simulink model "S4_ESC_Lab"  (R2025b)
settings: Solver=ode23t  StartTime=0.0  StopTime=inf  MaxStep=maxStep  RelTol=1e-4
values from neighbouring files (symbols this model uses):
  MF = [4 2.0 0.10 1.00]    [ABS_Utils.m]
undefined symbols (not defined in the file or in its folder): g, Jmax, Jmin, k, KiSlip, KpSlip, lambdaMax, lambdaMin, mode, mq, objectiveGain, Rw, stopV, Tmax, Tmin, Topen
libraries: nesl_utility x8, fl_lib x7, simulink x2, slctrl_adaptive x1, sdl_lib x1
settings Model: Creator=leffe  LastModifiedBy=leffe
settings OptimizationCC: BlockReduction=off  OptimizeBlockIOStorage=off

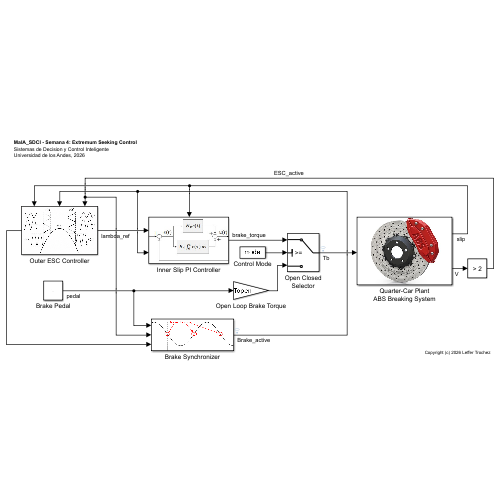
[thumbnail: Simulink's stored preview of the top-level diagram]
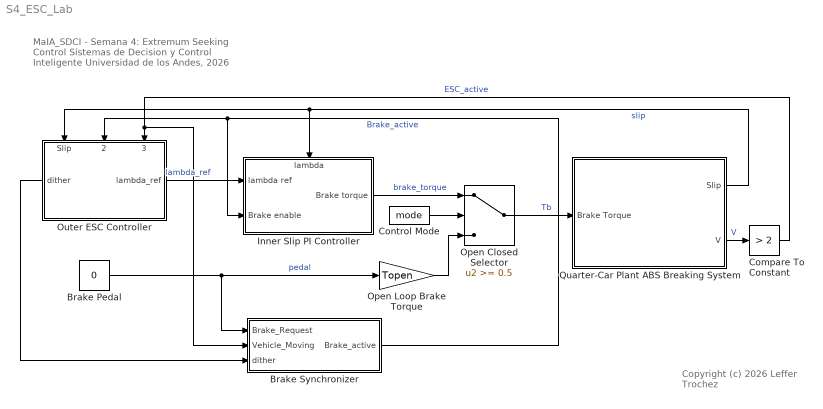
== system S4_ESC_Lab ==
  note: Copyright (c) 2026 Leffer Trochez
  note: MaIA_SDCI - Semana 4: Extremum Seeking Control
      | Sistemas de Decision y Control Inteligente
      | Universidad de los Andes, 2026
  Brake Pedal : Constant  Value=0  SampleTime=0
  Brake Synchronizer : Subsystem
      mask Display: image('hit crossing.png');
  Compare To Constant : simulink/Logic and Bit Operations/Compare To Constant  relop=>  const=2  OutDataTypeStr=boolean
  Control Mode : Constant  Value=mode
  Inner Slip PI Controller : Subsystem
      settings: PortSchema="{\"entries\":[{\"content\":{\"sides\":[{\"content\":{\"connectorIds\":[\"In1\",\"In2\"]},\"type\":\"ConnectorPlacement.EquallySpacedRectSide\",\"uuid\":\"2d8152cb-e1e7-4cbd-90d9-1ad452f9118c\"},{\"content\":{\"connectorIds\":[\"Out1\"],\"side\":\"RIGHT\"},\"type\":\"ConnectorPlacement.EquallySpacedRectSide\",\"uuid\":\"1543b6c9-e8db-48f7-9c77-f5e8a9c4fad1\"},{\"content\":{\"connectorIds\":[\"In3\"],\"side\":\"TOP\"},\"type\":\"ConnectorPlacement.EquallySpacedRectSide\",\"uuid\":\"3b9f2303-2b56-4e0e-9eaf-6ad78f3600f9\"}]},\"type\":\"ConnectorPlacement.EquallySpacedConnector\",\"uuid\":\"5e2a5701-87ef-4f6c-be32-195e55163038\"}],\"packageUris\":[\"http://schema.mathworks.com/mf0/Connector/R2020b\"],\"version\":\"1.0\"}"
      mask Display: image('PI.jpg');
  Open Closed Selector : Switch  Threshold=0.5  SaturateOnIntegerOverflow=off  InputSameDT=off
  Open Loop Brake Torque : Gain  Gain=Topen
  Outer ESC Controller : Subsystem
      settings: PortSchema="{\"entries\":[{\"content\":{\"sides\":[{\"content\":{\"connectorIds\":[\"Out2\"]},\"type\":\"ConnectorPlacement.EquallySpacedRectSide\",\"uuid\":\"31de49aa-46d4-4a9a-8690-efbb2b420d0d\"},{\"content\":{\"connectorIds\":[\"Out1\"],\"side\":\"RIGHT\"},\"type\":\"ConnectorPlacement.EquallySpacedRectSide\",\"uuid\":\"18edca33-0aae-4427-96c8-3219eae31a8b\"},{\"content\":{\"connectorIds\":[\"In1\",\"In2\",\"In3\"],\"side\":\"TOP\"},\"type\":\"ConnectorPlacement.EquallySpacedRectSide\",\"uuid\":\"43769023-76ac-4312-8342-8169355bc34d\"}]},\"type\":\"ConnectorPlacement.EquallySpacedConnector\",\"uuid\":\"6a090688-03d4-4148-bdef-ff5198eebe00\"}],\"packageUris\":[\"http://schema.mathworks.com/mf0/Connector/R2020b\"],\"version\":\"1.0\"}"
      mask Display: image('ESC.png');
  Quarter-Car Plant ABS Breaking System : Subsystem
      mask Display: image('ABS.jpg');
  wires:
  Brake Pedal/1 -> Brake Synchronizer/1(Brake_Request), Open Loop Brake Torque/1  "pedal"
  Inner Slip PI Controller/1(Brake torque) -> Open Closed Selector/1  "brake_torque"
  Quarter-Car Plant ABS Breaking System/1(Slip) -> Outer ESC Controller/1(Slip), Inner Slip PI Controller/3(lambda)  "slip"
  Open Loop Brake Torque/1 -> Open Closed Selector/3
  Control Mode/1 -> Open Closed Selector/2
  Open Closed Selector/1 -> Quarter-Car Plant ABS Breaking System/1(Brake Torque)  "Tb"
  Outer ESC Controller/1(lambda_ref) -> Inner Slip PI Controller/1(lambda ref)  "lambda_ref"
  Quarter-Car Plant ABS Breaking System/2(V) -> Compare To Constant/1  "V"
  Compare To Constant/1 -> Outer ESC Controller/3(ESC_active), Brake Synchronizer/2(Vehicle_Moving)  "ESC_active"
  Brake Synchronizer/1(Brake_active) -> Inner Slip PI Controller/2(Brake enable), Outer ESC Controller/2(Brake_active)  "Brake_active"
  Outer ESC Controller/2(dither) -> Brake Synchronizer/3(dither)

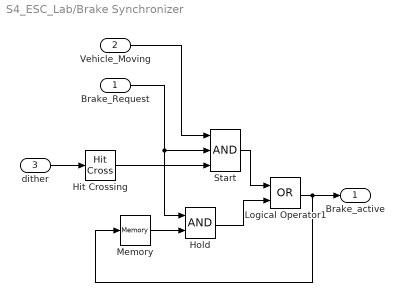
== system S4_ESC_Lab/Brake Synchronizer ==
  Brake_Request : Inport
  Vehicle_Moving : Inport  Port=2
  dither : Inport  Port=3
  Hit Crossing : HitCross  HitCrossingDirection=rising
  Hold : Logic  AllPortsSameDT=off  OutDataTypeStr=boolean
  Logical Operator1 : Logic  Operator=OR  AllPortsSameDT=off  OutDataTypeStr=boolean
  "Memory " : Memory
  Start : Logic  Inputs=3  AllPortsSameDT=off  OutDataTypeStr=boolean
  Brake_active : Outport
  wires:
  dither/1 -> Hit Crossing/1
  Brake_Request/1 -> Hold/1, Start/2
  Vehicle_Moving/1 -> Start/1
  Hit Crossing/1 -> Start/3
  "Memory "/1 -> Hold/2
  Start/1 -> Logical Operator1/1
  Hold/1 -> Logical Operator1/2
  Logical Operator1/1 -> "Memory "/1, Brake_active/1

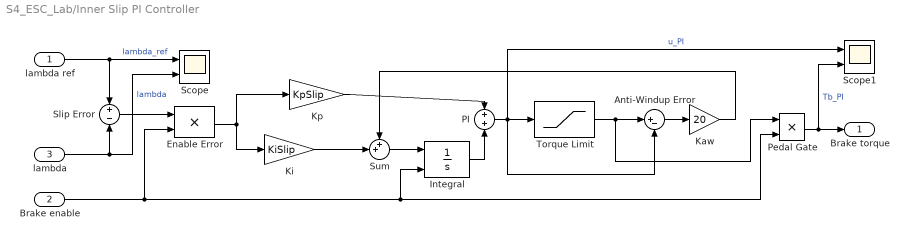
== system S4_ESC_Lab/Inner Slip PI Controller ==
  lambda ref : Inport
  Brake enable : Inport  Port=2
  lambda : Inport  Port=3
  Anti-Windup Error : Sum  Inputs=|+-
  Enable Error : Product  Inputs=**
  Integral : Integrator  ExternalReset=falling  LimitOutput=on  UpperSaturationLimit=Tmax  LowerSaturationLimit=0
  Kaw : Gain  Gain=20
  Ki : Gain  Gain=KiSlip
  Kp : Gain  Gain=KpSlip
  PI : Sum
  Pedal Gate : Product  Inputs=**
  Scope : Scope  NumInputPorts=2
      settings: ActiveDisplayYMinimum=-0.024789664527761449  ActiveDisplayYMaximum=0.22310698074985311
  Scope1 : Scope  NumInputPorts=2
      settings: ActiveDisplayYMinimum=-525.00598935884784  ActiveDisplayYMaximum=4725.0539042296314
  Slip Error : Sum  Inputs=+-
  Sum : Sum  Inputs=++|
  Torque Limit : Saturate  UpperLimit=Tmax  LowerLimit=Tmin
  Brake torque : Outport
  wires:
  Slip Error/1 -> Enable Error/1
  Brake enable/1 -> Enable Error/2, Pedal Gate/2, Integral/2
  Enable Error/1 -> Kp/1, Ki/1
  Kp/1 -> PI/1
  Integral/1 -> PI/2
  PI/1 -> Anti-Windup Error/2, Scope1/1, Torque Limit/1  "u_PI"
  Pedal Gate/1 -> Brake torque/1, Scope1/2  "Tb_PI"
  lambda ref/1 -> Slip Error/1, Scope/1  "lambda_ref"
  lambda/1 -> Slip Error/2, Scope/2  "lambda"
  Torque Limit/1 -> Anti-Windup Error/1, Pedal Gate/1
  Anti-Windup Error/1 -> Kaw/1
  Sum/1 -> Integral/1
  Ki/1 -> Sum/2
  Kaw/1 -> Sum/1

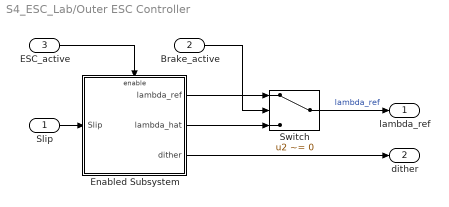
== system S4_ESC_Lab/Outer ESC Controller ==
  Slip : Inport
  Brake_active : Inport  Port=2
  ESC_active : Inport  Port=3
  "Enabled Subsystem " : Subsystem  TreatAsAtomicUnit=on
  Switch : Switch  Criteria=u2 ~= 0  SaturateOnIntegerOverflow=off  InputSameDT=off
  lambda_ref : Outport
  dither : Outport  Port=2
  wires:
  Slip/1 -> "Enabled Subsystem "/1(Slip)
  "Enabled Subsystem "/1(lambda_ref) -> Switch/1
  Brake_active/1 -> Switch/2
  "Enabled Subsystem "/2(lambda_hat) -> Switch/3
  Switch/1 -> lambda_ref/1  "lambda_ref"
  "Enabled Subsystem "/3(dither) -> dither/1
  ESC_active/1 -> "Enabled Subsystem "/Enable

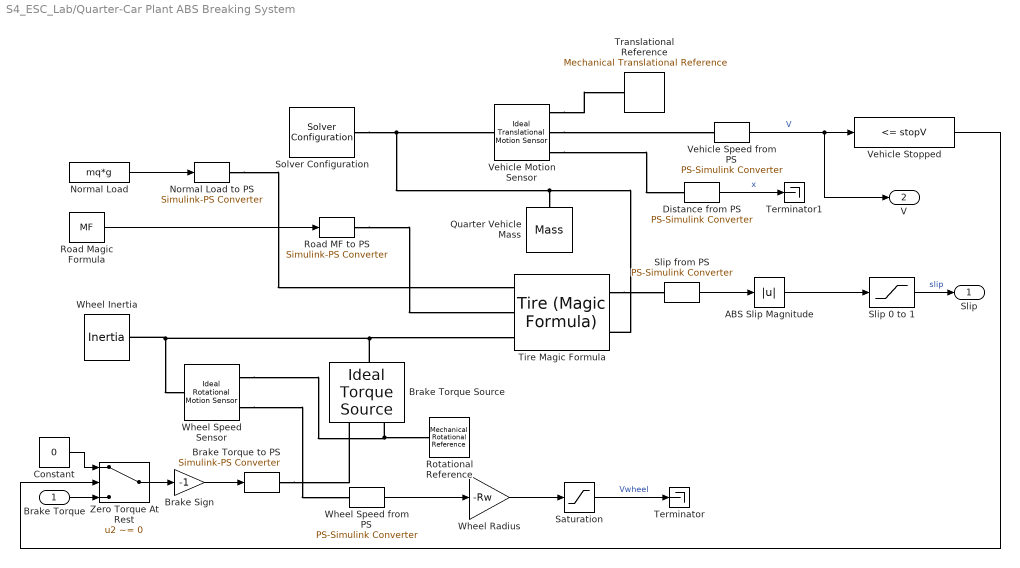
== system S4_ESC_Lab/Quarter-Car Plant ABS Breaking System ==
  Brake Torque : Inport
  ABS Slip Magnitude : Abs  SaturateOnIntegerOverflow=off
  Brake Sign : Gain  Gain=-1
  Brake Torque Source : fl_lib/Mechanical/Mechanical Sources/Ideal Torque Source
  Brake Torque to PS : nesl_utility/Simulink-PS Converter  PhysicalDomain=network_engine_domain  SubClassName=ps_input  LeftPortType=input  RightPortType=output  PseudoPeriodic=off  Frequencies=[]  NoiseDistribution=none  NoiseParameters=[]  Unit=N*m  AffineConversion=off  FilteringAndDerivatives=provide  SimscapeFilterOrder=1  InputFilterTimeConstant=0.001  UdotUserProvided=0
  Constant : Constant  Value=0
  Distance from PS : nesl_utility/PS-Simulink Converter  PhysicalDomain=network_engine_domain  SubClassName=ps_output  LeftPortType=input  RightPortType=output  PseudoPeriodic=off  Frequencies=[]  VectorFormat=inherit  Unit=m  AffineConversion=off
  Normal Load : Constant  Value=mq*g
  Normal Load to PS : nesl_utility/Simulink-PS Converter  PhysicalDomain=network_engine_domain  SubClassName=ps_input  LeftPortType=input  RightPortType=output  PseudoPeriodic=off  Frequencies=[]  NoiseDistribution=none  NoiseParameters=[]  Unit=N  AffineConversion=off  FilteringAndDerivatives=provide  SimscapeFilterOrder=1  InputFilterTimeConstant=0.001  UdotUserProvided=0
  Quarter Vehicle Mass : fl_lib/Mechanical/Translational Elements/Mass  mass=mq kg  num_ports=foundation.enum.numPorts2.one  v_specify=on  v_priority=High  v=v0 m/s  v_nominal_specify=off  v_nominal_value=1  v_nominal_unit=m/s  f_specify=off  f_priority=None  f=0 N  f_nominal_specify=off  f_nominal_value=1  f_nominal_unit=N
  Road MF to PS : nesl_utility/Simulink-PS Converter  PhysicalDomain=network_engine_domain  SubClassName=ps_input  LeftPortType=input  RightPortType=output  PseudoPeriodic=off  Frequencies=[]  NoiseDistribution=none  NoiseParameters=[]  Unit=1  AffineConversion=off  FilteringAndDerivatives=provide  SimscapeFilterOrder=1  InputFilterTimeConstant=0.001  UdotUserProvided=0
  Road Magic Formula : Constant  Value=MF
  Rotational Reference : fl_lib/Mechanical/Rotational Elements/Mechanical Rotational Reference
  Saturation : Saturate  UpperLimit=0  LowerLimit=-inf
  Slip 0 to 1 : Saturate  UpperLimit=1  LowerLimit=0
  Slip from PS : nesl_utility/PS-Simulink Converter  PhysicalDomain=network_engine_domain  SubClassName=ps_output  LeftPortType=input  RightPortType=output  PseudoPeriodic=off  Frequencies=[]  VectorFormat=inherit  Unit=1  AffineConversion=off
  Solver Configuration : nesl_utility/Solver Configuration  PhysicalDomain=network_engine_domain  SubClassName=solver  LeftPortType=input  RightPortType=generic  Tones=[]  Harmonics=[]  SimulateNoise=off  Profile=off  UseLocalSampling=off  EnableSwitchedLinearOptims=on  FrequencyDomain=off  UseCCode=off  RelTol=0.001  AbsTol=0.001  MinStep=1e-09  ToWorkspace=off  RevertToSquareIcSolve=off  NumHomotopyIterations=100  PhasorMode=off  PhasorModeNumHarmonics=1  ConsistencySolver=NEWTON_XTOL_AFTER_FTOL  IndexReductionMethod=DerivativeReplacement  DoDC=off  ResidualTolerance=1e-09  ConsistencyTolSource=GLOBAL  ConsistencyAbsTol=0.001  ConsistencyRelTol=0.001  ConsistencyTolFactor=0.001  UseLocalSolver=off  LocalSolverChoice=NE_BACKWARD_EULER_ADVANCER  ResolveIndetEquations=on  FunctionEvalNumThread=1  LocalSolverSampleTime=0.001  DoFixedCost=off  MaxNonlinIter=3  MaxModeIter=2  ComputeImpulses=off  ImpulseIterations=2  LinearAlgebra=auto  LinearAlgebraNumThread=0  EquationFormulation=NE_TIME_EF  DelaysMemoryBudget=1024  AutomaticFiltering=on  FilteringTimeConstant=0.001  PartitionStorageMethod=AS_NEEDED  PartitionMemoryBudget=1024  PartitionMethod=ROBUST  MultibodyUseLocalSolver=off  MultibodyLocalSolverChoice=ODE1  MultibodyLocalSolverSampleTime=0.001
  Terminator : Terminator
  Terminator1 : Terminator
  Tire Magic Formula : sdl_lib/Tires & Vehicles/Tire (Magic Formula)  parameterization=sdl.enum.magic_tire_model.PS  F_z1=3000 N  F_x1=3500 N  kappa1=10  B_m=10  C_m=1.9  D_m=1  E_m=0.97  fz0=4000 N  p_Cx=1.685  p_Dx=[1.21, -.037]  p_Ex=[.344, .095, -.02, 0]  p_Kx=[21.51, -.163, .245]  p_Hx=[-.002, .002]  p_Vx=[0, 0]  rolling_radius_model=sdl.enum.RollingRadiusParameterization.Constant  r_e=Rw m  r_0=0.3 m  breff=8.39  dreff=0.26  freff=0.074  q_re0=0.99  q_v1=0.008  longvl=17 m/s  cz=5e5 N/m  model_resistance=0  resistance_model=sdl.enum.rollingResistanceParameterization.constant  coeff=0.015  p_tire=250e3 Pa  alpha=-0.003  beta=0.97  coeff_a=84e-4  coeff_b=6.2e-4 s/m  coeff_c=1.6e-4 s^2/m^2  p_tire0=240e3 Pa  fz0_resistance=4000 N  vH0=16 m/s  q_Sy=[.0082, 0, .0014, .001, 0, 0, 1.08, -.5]  v_thr=0.001 m/s  enable_scaling_coefficients=false  lfzO=1  lcx=1  lmux=1  lex=1  lkx=1  lhx=1  lvx=1  lmy=1  model_compliance=0  stiffness=1e6 N/m  damping=1000 N*s/m  model_inertia=0  inertia=1 kg*m^2  initial_velocity=0 rad/s  vxlow=1 m/s  v_tr_thr=0.1 m/s  kpumin=-1.5  kpumax=1.5
      settings: InternalSimscapePortConfiguration="{\"Bottom\":[],\"Left\":[{\"id\":\"N\",\"label\":\"N\",\"type\":\"input\"},{\"id\":\"M\",\"label\":\"M\",\"type\":\"input\"},{\"id\":\"A\",\"label\":\"A\",\"type\":\"foundation.mechanical.rotational.rotational\"}],\"Right\":[{\"id\":\"S\",\"label\":\"S\",\"type\":\"output\"},{\"id\":\"H\",\"label\":\"H\",\"type\":\"foundation.mechanical.translational.translational\"}],\"Top\":[]}"
  Translational Reference : fl_lib/Mechanical/Translational Elements/Mechanical Translational Reference
  Vehicle Motion Sensor : fl_lib/Mechanical/Mechanical Sensors/Ideal Translational Motion Sensor  reference=foundation.enum.MeasurementReference.difference  acceleration_port=false  velocity_port=true  position_port=true  offset=0 m
  Vehicle Speed from PS : nesl_utility/PS-Simulink Converter  PhysicalDomain=network_engine_domain  SubClassName=ps_output  LeftPortType=input  RightPortType=output  PseudoPeriodic=off  Frequencies=[]  VectorFormat=inherit  Unit=m/s  AffineConversion=off
  Vehicle Stopped : simulink/Logic and Bit Operations/Compare To Constant  relop=<=  const=stopV  OutDataTypeStr=boolean
  Wheel Inertia : fl_lib/Mechanical/Rotational Elements/Inertia  inertia=Jw kg*m^2  num_ports=foundation.enum.numPorts2.one  w_specify=on  w_priority=High  w=w0 rad/s  w_nominal_specify=off  w_nominal_value=1  w_nominal_unit=rad/s  t_specify=off  t_priority=None  t=0 N*m  t_nominal_specify=off  t_nominal_value=1  t_nominal_unit=N*m
  Wheel Radius : Gain  Gain=-Rw
  Wheel Speed Sensor : fl_lib/Mechanical/Mechanical Sensors/Ideal Rotational Motion Sensor  reference=foundation.enum.MeasurementReference.difference  acceleration_port=false  velocity_port=true  position_port=false  wrap_angle=false  offset=0 rad
      settings: InternalSimscapePortConfiguration="{\"Bottom\":[],\"Left\":[{\"id\":\"R\",\"label\":\"R\",\"type\":\"foundation.mechanical.rotational.rotational\"}],\"Right\":[{\"id\":\"C\",\"label\":\"C\",\"type\":\"foundation.mechanical.rotational.rotational\"},{\"id\":\"W\",\"label\":\"W\",\"type\":\"output\"}],\"Top\":[]}"
  Wheel Speed from PS : nesl_utility/PS-Simulink Converter  PhysicalDomain=network_engine_domain  SubClassName=ps_output  LeftPortType=input  RightPortType=output  PseudoPeriodic=off  Frequencies=[]  VectorFormat=inherit  Unit=rad/s  AffineConversion=off
  Zero Torque At Rest : Switch  Criteria=u2 ~= 0  SaturateOnIntegerOverflow=off  InputSameDT=off
  Slip : Outport
  V : Outport  Port=2
  wires:
  Normal Load/1 -> Normal Load to PS/1
  Road Magic Formula/1 -> Road MF to PS/1
  Wheel Speed from PS/1 -> Wheel Radius/1
  Slip from PS/1 -> ABS Slip Magnitude/1
  Distance from PS/1 -> Terminator1/1  "x"
  ABS Slip Magnitude/1 -> Slip 0 to 1/1
  Slip 0 to 1/1 -> Slip/1  "slip"
  Vehicle Speed from PS/1 -> V/1, Vehicle Stopped/1  "V"
  Vehicle Stopped/1 -> Zero Torque At Rest/2
  Constant/1 -> Zero Torque At Rest/1
  Brake Torque/1 -> Zero Torque At Rest/3
  Wheel Radius/1 -> Saturation/1
  Zero Torque At Rest/1 -> Brake Sign/1
  Brake Sign/1 -> Brake Torque to PS/1
  Saturation/1 -> Terminator/1  "Vwheel"
  connections:
  Brake Torque to PS/RConn1 -- Brake Torque Source/RConn1
  Wheel Speed Sensor/RConn1 -- Brake Torque Source/RConn2 -- Rotational Reference/LConn1
  Wheel Speed Sensor/RConn2 -- Wheel Speed from PS/LConn1
  Normal Load to PS/RConn1 -- Tire Magic Formula/LConn1
  Solver Configuration/RConn1 -- Tire Magic Formula/RConn2 -- Quarter Vehicle Mass/LConn1 -- Vehicle Motion Sensor/LConn1
  Road MF to PS/RConn1 -- Tire Magic Formula/LConn2
  Brake Torque Source/LConn1 -- Wheel Speed Sensor/LConn1 -- Wheel Inertia/LConn1 -- Tire Magic Formula/LConn3
  Vehicle Motion Sensor/RConn2 -- Vehicle Speed from PS/LConn1
  Vehicle Motion Sensor/RConn1 -- Translational Reference/LConn1
  Vehicle Motion Sensor/RConn3 -- Distance from PS/LConn1
  Tire Magic Formula/RConn1 -- Slip from PS/LConn1

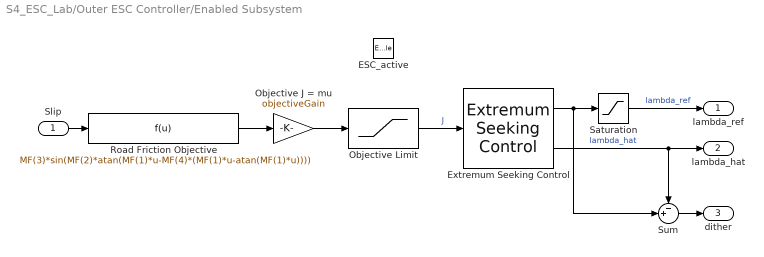
== system S4_ESC_Lab/Outer ESC Controller/Enabled Subsystem  ==
  Slip : Inport
  ESC_active : EnablePort
  " Saturation " : Saturate  UpperLimit=lambdaMax  LowerLimit=lambdaMin
  "Extremum Seeking Control " : slctrl_adaptive/Extremum Seeking Control  timeDomainStatus=Continuous time  SampleTime=0.1  IntegratorMethods=Forward Euler  paramCount=1  initialVal=lambda0  omega=omega  gain=k  demodAmp=demodAmp  demodPhase=demodPhase  modAmp=b  modPhase=modPhase  highPassEnable=on  highPassCutoff=wh  lowPassEnable=on  lowPassCutoff=wl  estimatedVarOn=on  HPFFreq=1  LPFFreq=2  SampleTimeVar=0
      settings: LibrarySourceBlock=slctrlblks/Adaptive Control/Extremum Seeking Control
  Objective J = mu : Gain  Gain=objectiveGain
  Objective Limit : Saturate  UpperLimit=Jmax  LowerLimit=Jmin
  Road Friction Objective : Fcn  Expr=MF(3)*sin(MF(2)*atan(MF(1)*u-MF(4)*(MF(1)*u-atan(MF(1)*u))))
  Sum : Sum  Inputs=-+|
  lambda_ref : Outport
  lambda_hat : Outport  Port=2
  dither : Outport  Port=3
  wires:
  "Extremum Seeking Control "/1 -> Sum/2, " Saturation "/1
  Road Friction Objective/1 -> Objective J = mu/1
  Slip/1 -> Road Friction Objective/1
  Objective Limit/1 -> "Extremum Seeking Control "/1  "J"
  " Saturation "/1 -> lambda_ref/1  "lambda_ref"
  "Extremum Seeking Control "/2 -> lambda_hat/1, Sum/1  "lambda_hat"
  Objective J = mu/1 -> Objective Limit/1
  Sum/1 -> dither/1
